simulink model "ModelDFix"  (R2018a)
settings: Solver=ode23  StartTime=0.0  StopTime=0.1  MaxStep=10e-6  RelTol=1e-3
libraries: powerlib x14
settings Model: Creator=ivank  LastModifiedBy=ivank
settings SolverCC: InitialStep=10e-8

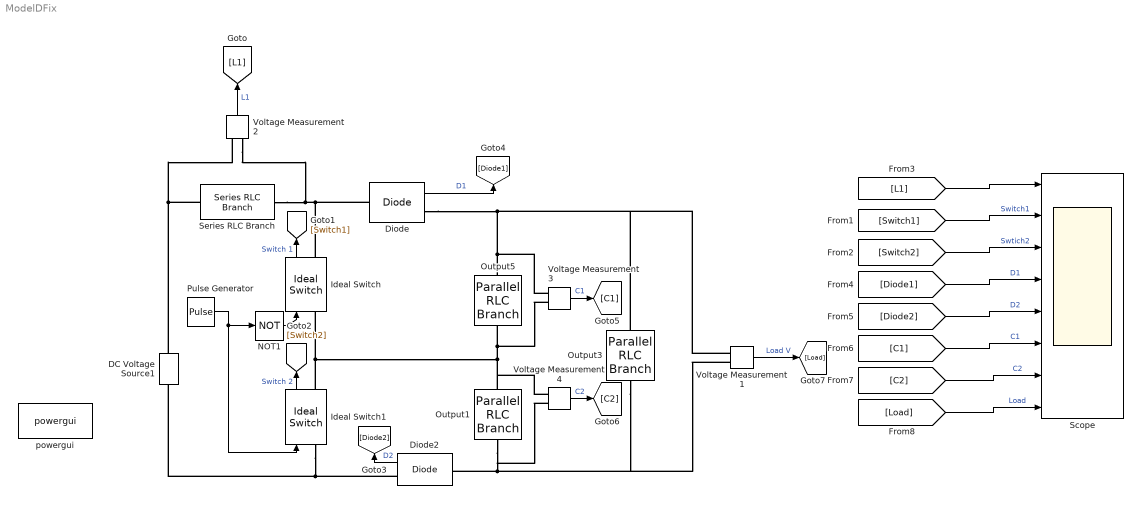
== system ModelDFix ==
  DC Voltage Source1 : powerlib/Electrical Sources/DC Voltage Source  Amplitude=10  Measurements=Voltage
  Diode : powerlib/Power Electronics/Diode  Ron=0.001  Lon=0  Vf=0.8  IC=0  UseSnubber=0  Rs=500  Cs=250e-9  Measurements=on
  Diode2 : powerlib/Power Electronics/Diode  Ron=0.001  Lon=0  Vf=0.8  IC=0  UseSnubber=0  Rs=500  Cs=250e-9  Measurements=on
  Ideal Switch : powerlib/Power Electronics/Ideal Switch  Ron=0.001  Lon=0  IC=0  Rs=1e5  Cs=inf  Measurements=on
  Ideal Switch1 : powerlib/Power Electronics/Ideal Switch  Ron=0.001  Lon=0  IC=0  Rs=1e5  Cs=inf  Measurements=on
  NOT1 : Logic  Operator=NOT  IconShape=distinctive  AllPortsSameDT=off  OutDataTypeStr=boolean
  Output1 : powerlib/Elements/Parallel RLC Branch  LConnTagsString=a  RConnTagsString=__new0  BranchType=C  Resistance=7.225  Inductance=1e-3  SetiL0=off  InitialCurrent=0  Capacitance=220e-6  Setx0=off  InitialVoltage=0  Measurements=Branch voltage and current
  Output3 : powerlib/Elements/Parallel RLC Branch  LConnTagsString=a  RConnTagsString=__new0  BranchType=R  Resistance=225  Inductance=1e-3  SetiL0=off  InitialCurrent=0  Capacitance=100*10e-6  Setx0=off  InitialVoltage=0  Measurements=Branch voltage and current
  Output5 : powerlib/Elements/Parallel RLC Branch  LConnTagsString=a  RConnTagsString=__new0  BranchType=C  Resistance=7.225  Inductance=1e-3  SetiL0=off  InitialCurrent=0  Capacitance=220e-6  Setx0=off  InitialVoltage=0  Measurements=Branch voltage and current
  Pulse Generator : DiscretePulseGenerator  PulseType=Time based  Period=1/50000  PulseWidth=50  VectorParams1D=off
  Scope : Scope  NumInputPorts=8
  Series RLC Branch : powerlib/Elements/Series RLC Branch  LConnTagsString=__new0  RConnTagsString=__new0  BranchType=L  Resistance=.01  Inductance=150e-6  SetiL0=off  InitialCurrent=0  Capacitance=1e-6  Setx0=off  InitialVoltage=0  Measurements=Branch voltage and current
  Voltage Measurement{1..4} (4 alike) : powerlib/Measurements/Voltage Measurement  PhasorSimulation=off  OutputType=Complex  PSBequivalent=0
  powergui : powerlib/powergui  Priority=1  SimulationMode=Continuous  SampleTime=50e-6  frequency=60  Iterations=50  frequencyindice=0  Pbase=100e6  ErrMax=1e-4  UnitsV=kV  UnitsW=MW  buscounter=0  FunctionMessages=off  echomessages=off  EnableUseOfTLC=off  CurrentSourceSwitches=off  DisableSnubberDevices=off  DisableRonSwitches=off  DisableVfSwitches=off  DisplayEquations=off  SolverType=Tustin/Backward Euler (TBE)  Interpol=off  ExternalGateDelay=off  methode=off  Ts=100  x0status=blocks  SPID=on  SwTol=0  HookPort=off  RestoreLinks=warning  ResistiveCurrentMeasurement=off  Frange=[0:2:500]  Ylog=off  Xlog=on  ShowGrid=off  save=off  variable=ZData  structure=0  ZoomFFT=off  StartTime=0.0  cycles=1  DisplayStyle=1  fundamental=60  FreqAxis=off  MaxFrequency=1000  frequencyindicesteady=1  RmsSteady=1  display=off
  wires:
  Pulse Generator/1 -> Ideal Switch1/1, NOT1/1
  Voltage Measurement2/1 -> [L1]  "L1"
  [L1] -> Scope/1
  Ideal Switch/1 -> [Switch1]  "Switch 1"
  Ideal Switch1/1 -> [Switch2]  "Switch 2"
  Diode2/1 -> [Diode2]  "D2"
  Diode/1 -> [Diode1]  "D1"
  [Switch1] -> Scope/2  "Switch1"
  [Switch2] -> Scope/3  "Swtich2"
  [Diode1] -> Scope/4  "D1"
  [Diode2] -> Scope/5  "D2"
  [C1] -> Scope/6  "C1"
  [C2] -> Scope/7  "C2"
  [Load] -> Scope/8  "Load"
  Voltage Measurement3/1 -> [C1]  "C1"
  Voltage Measurement4/1 -> [C2]  "C2"
  Voltage Measurement1/1 -> [Load]  "Load V"
  NOT1/1 -> Ideal Switch/1
  connections:
  Diode2/RConn1 -- Ideal Switch1/LConn1 -- DC Voltage Source1/LConn1
  DC Voltage Source1/RConn1 -- Voltage Measurement2/LConn2 -- Series RLC Branch/LConn1
  Output5/LConn1 -- Voltage Measurement3/LConn1 -- Voltage Measurement1/LConn1 -- Output3/LConn1 -- Diode/RConn1
  Output3/RConn1 -- Voltage Measurement1/LConn2 -- Voltage Measurement4/LConn2 -- Output1/RConn1 -- Diode2/LConn1
  Ideal Switch/RConn1 -- Diode/LConn1 -- Voltage Measurement2/LConn1 -- Series RLC Branch/RConn1
  Ideal Switch1/RConn1 -- Ideal Switch/LConn1 -- Voltage Measurement4/LConn1 -- Output1/LConn1 -- Voltage Measurement3/LConn2 -- Output5/RConn1
